simulink model "euler_kinematic"  (R2018b)
settings: Solver=ode113  StartTime=0.0  StopTime=1000  RelTol=1e-3
settings Model: Creator=Stefano  LastModifiedBy=Stefano
settings SolverCC: DecoupledContinuousIntegration=on  MinimalZcImpactIntegration=on
settings DebuggingCC: LibraryContextMissingDiagnostic=none
settings SFSimCC: SimUseLocalCustomCode=off
settings RTWCC: RTWUseLocalCustomCode=off

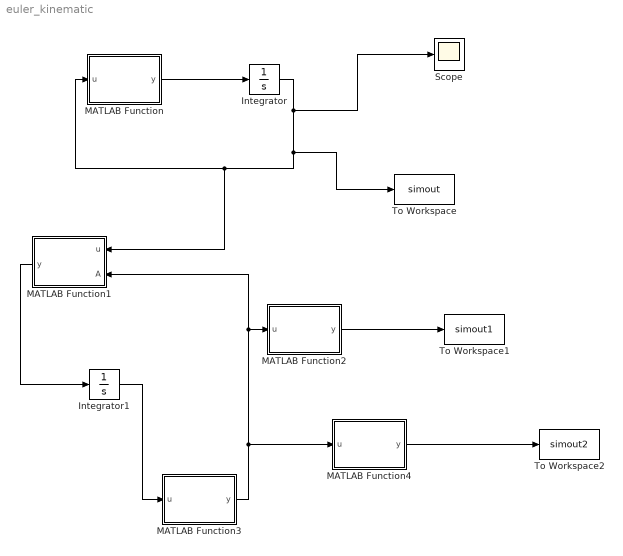
== system euler_kinematic ==
  Integrator : Integrator  InitialCondition=[0.01; 0.01; 15*pi/180]
  Integrator1 : Integrator  InitialCondition=[1 0 0;0 1 0;0 0 1]
  MATLAB Function : MATLAB Function  TreatAsAtomicUnit=on
  MATLAB Function1 : MATLAB Function  TreatAsAtomicUnit=on
  MATLAB Function2 : MATLAB Function  TreatAsAtomicUnit=on
  MATLAB Function3 : MATLAB Function  TreatAsAtomicUnit=on
  MATLAB Function4 : MATLAB Function  TreatAsAtomicUnit=on
  Scope : Scope
  To Workspace : ToWorkspace  VariableName=simout  SaveFormat=Timeseries  SampleTime=-1
  To Workspace1 : ToWorkspace  VariableName=simout1  SaveFormat=Timeseries  SampleTime=-1
  To Workspace2 : ToWorkspace  VariableName=simout2  SampleTime=-1
  wires:
  MATLAB Function/1(y) -> Integrator/1
  Integrator/1 -> Scope/1, To Workspace/1, MATLAB Function1/1(u), MATLAB Function/1(u)
  MATLAB Function1/1(y) -> Integrator1/1
  MATLAB Function2/1(y) -> To Workspace1/1
  Integrator1/1 -> MATLAB Function3/1(u)
  MATLAB Function3/1(y) -> MATLAB Function2/1(u), MATLAB Function1/2(A), MATLAB Function4/1(u)
  MATLAB Function4/1(y) -> To Workspace2/1

== matlab function euler_kinematic/MATLAB Function1 ==
  data: u input; y output; A input
function y = fcn(u,A)

W=[0 -u(3) u(2);u(2) 0 -u(1);-u(2) u(1) 0];
Adot=-W*A;
y=Adot;
end

== matlab function euler_kinematic/MATLAB Function ==
  data: u input; y output
function y = fcn(u)
%First laboratory

%Datas
Ix=0.01;
Iy=0.05;
Iz=0.07;

omx=u(1);
omy=u(2);
omz=u(3);

%Formula
omxdot=(Iy-Iz)/Ix*omy*omz;
omydot=(Iz-Ix)/Iy*omx*omz;
omzdot=(Ix-Iy)/Iz*omy*omx;

y=[omxdot; omydot; omzdot];

u=y;

end

== matlab function euler_kinematic/MATLAB Function2 ==
  data: u input; y output
function y = fcn(u)

t=trace(eye(3)-(u')*u);
y=t;

end

== matlab function euler_kinematic/MATLAB Function3 ==
  data: u input; y output
function y = fcn(u)

t=abs(trace(eye(3)-u'*u));
while t>0.00000001
    A=(1.5)*u-u*u'*0.5*u;
    t=abs(trace(eye(3)-A'*A));
    u=A;
end

y=u;
end

== matlab function euler_kinematic/MATLAB Function4 ==
  data: u input; y output
function y = fcn(u)

y=u'*[0 0 1]';

end
